simulink library "aero_lib"  (Simulink 7.2)
settings: Solver=ode45  SolverMode=SingleTasking  StartTime=0.0  StopTime=10.0  RelTol=1e-3
undefined symbols (not defined in the file or in its folder): b, symmetric_aero_on
libraries: GTM_aerolib x3, aero_lib x1, aeroutilslib x1, simulink x1
settings Model: Creator=amurch  LastModifiedBy=la1032aw  ExtModeAutoUpdateStatusClock=off

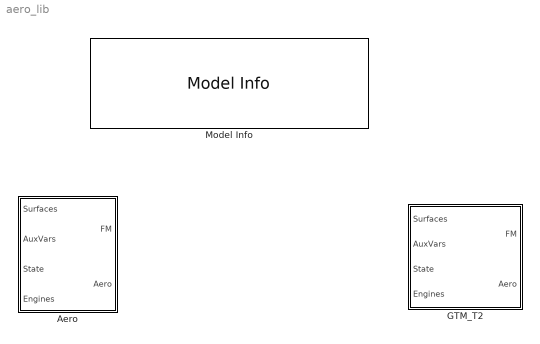
== system aero_lib ==
  Aero : Subsystem  BlockChoice=GTM_T2
      settings: TemplateBlock=self  MemberBlocks=GTM_T2
  GTM_T2 : Subsystem
  Model Info : simulink/Model-Wide Utilities/Model Info  SystemSampleTime=-1  InitialBlockCM=None  BlockCM=None  Frame=on  DisplayStringWithTags=|  HorizontalTextAlignment=Center  LeftAlignmentValue=0.5  SourceBlockDiagram=aero_lib  TagMaxNumber=20
      | AirSTAR Aerodynamic Model Library
      | %<ModelVersion>
      | Last modified by %<LastModifiedBy> on %<LastModificationDate>

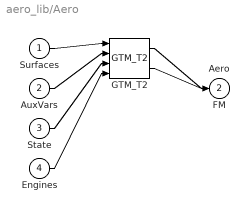
== system aero_lib/Aero ==
  Surfaces : Inport  OutDataType=sfix(16)  OutScaling=2^0
  AuxVars : Inport  Port=2  OutDataType=sfix(16)  OutScaling=2^0
  State : Inport  Port=3  OutDataType=sfix(16)  OutScaling=2^0
  Engines : Inport  Port=4  OutDataType=sfix(16)  OutScaling=2^0
  GTM_T2 : aero_lib/GTM_T2  SystemSampleTime=-1
  FM : Outport  OutDataType=sfix(16)  OutScaling=2^0
  Aero : Outport  Port=2  OutDataType=sfix(16)  OutScaling=2^0
  wires:
  Surfaces/1 -> GTM_T2/1
  AuxVars/1 -> GTM_T2/2
  State/1 -> GTM_T2/3
  Engines/1 -> GTM_T2/4
  GTM_T2/1 -> FM/1
  GTM_T2/2 -> Aero/1

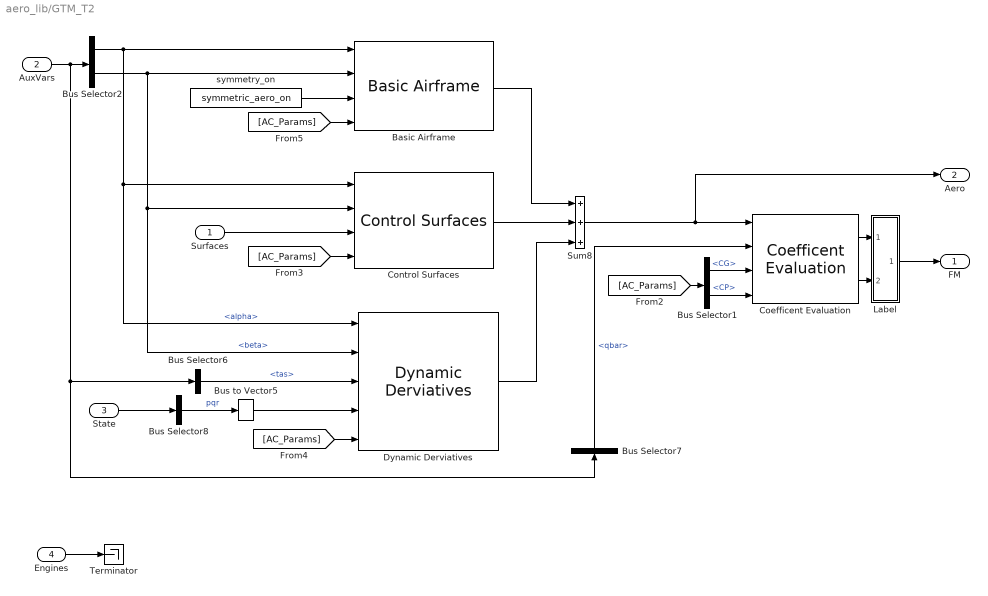
== system aero_lib/GTM_T2 ==
  Surfaces : Inport  OutDataType=sfix(16)  OutScaling=2^0
  AuxVars : Inport  Port=2  OutDataType=sfix(16)  OutScaling=2^0
  State : Inport  Port=3  OutDataType=sfix(16)  OutScaling=2^0
  Engines : Inport  Port=4  OutDataType=sfix(16)  OutScaling=2^0
  Basic Airframe : GTM_aerolib/Basic Airframe  SystemSampleTime=-1
  Bus Selector1 : BusSelector  OutputSignals=CG,CP
  Bus Selector2 : BusSelector  OutputSignals=alpha,beta
  Bus Selector6 : BusSelector  OutputSignals=tas
  Bus Selector7 : BusSelector  Orientation=up  OutputSignals=qbar
  Bus Selector8 : BusSelector  OutputSignals=pb,qb,rb  OutputAsBus=on
  Bus to Vector5 : BusToVector
  Coefficent Evaluation : aeroutilslib/Coefficent Evaluation  SystemSampleTime=-1  b=b  cbar=Cbar  Sref=S
  Control Surfaces : GTM_aerolib/Control Surfaces  SystemSampleTime=-1
  Dynamic Derviatives : GTM_aerolib/Dynamic Derviatives  SystemSampleTime=-1
  Label : Subsystem
  Sum8 : Sum  Inputs=+++  OutDataType=sfix(16)  OutScaling=2^0  SaturateOnIntegerOverflow=on  InputSameDT=on  OutDataTypeStr=Inherit: Same as first input
  Terminator : Terminator
  symmetry_on : Constant  Value=symmetric_aero_on  OutDataType=sfix(16)  OutScaling=2^0
  FM : Outport  OutDataType=sfix(16)  OutScaling=2^0
  Aero : Outport  Port=2  OutDataType=sfix(16)  OutScaling=2^0
  wires:
  Surfaces/1 -> Control Surfaces/3
  symmetry_on/1 -> Basic Airframe/3
  Bus Selector1/2 -> Coefficent Evaluation/4  "<CP>"
  [AC_Params] -> Bus Selector1/1
  Bus Selector1/1 -> Coefficent Evaluation/3  "<CG>"
  Coefficent Evaluation/2 -> Label/2(Im)
  Coefficent Evaluation/1 -> Label/1(If)
  Sum8/1 -> Coefficent Evaluation/1, Aero/1
  Bus Selector7/1 -> Coefficent Evaluation/2  "<qbar>"
  Label/1(O) -> FM/1
  AuxVars/1 -> Bus Selector7/1, Bus Selector6/1, Bus Selector2/1
  Bus Selector2/1 -> Control Surfaces/1, Dynamic Derviatives/1, Basic Airframe/1  "<alpha>"
  Bus Selector2/2 -> Control Surfaces/2, Dynamic Derviatives/2, Basic Airframe/2  "<beta>"
  State/1 -> Bus Selector8/1
  Dynamic Derviatives/1 -> Sum8/3
  Control Surfaces/1 -> Sum8/2
  Basic Airframe/1 -> Sum8/1
  Engines/1 -> Terminator/1
  Bus Selector8/1 -> Bus to Vector5/1  "pqr"
  [AC_Params] -> Basic Airframe/4
  [AC_Params] -> Control Surfaces/4
  Bus Selector6/1 -> Dynamic Derviatives/3  "<tas>"
  Bus to Vector5/1 -> Dynamic Derviatives/4
  [AC_Params] -> Dynamic Derviatives/5

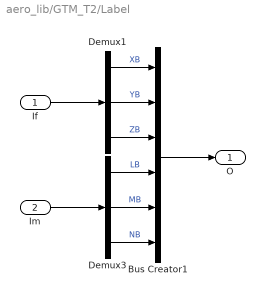
== system aero_lib/GTM_T2/Label ==
  If : Inport  OutDataType=sfix(16)  OutScaling=2^0
  Im : Inport  Port=2  OutDataType=sfix(16)  OutScaling=2^0
  Bus Creator1 : BusCreator  Inputs=6
  Demux1 : Demux  Outputs=3
  Demux3 : Demux  Outputs=3
  O : Outport  OutDataType=sfix(16)  OutScaling=2^0
  wires:
  Im/1 -> Demux3/1
  Demux3/3 -> Bus Creator1/6  "NB"
  Demux3/2 -> Bus Creator1/5  "MB"
  Demux3/1 -> Bus Creator1/4  "LB"
  Demux1/3 -> Bus Creator1/3  "ZB"
  Demux1/2 -> Bus Creator1/2  "YB"
  Demux1/1 -> Bus Creator1/1  "XB"
  If/1 -> Demux1/1
  Bus Creator1/1 -> O/1
